simulink model "TaliRo_monitoring_subsytem"  (R2019b)
settings: Solver=VariableStepAuto  StartTime=0.0  StopTime=10.0  RelTol=1e-3
undefined symbols (not defined in the file): nb_rooms, nb_step_to_fifteen_min, nb_step_to_one_h, nb_step_to_thirty_min
libraries: S_TaLiRo x6, dspstat3 x6
settings Model: Creator=tong  LastModifiedBy=pat

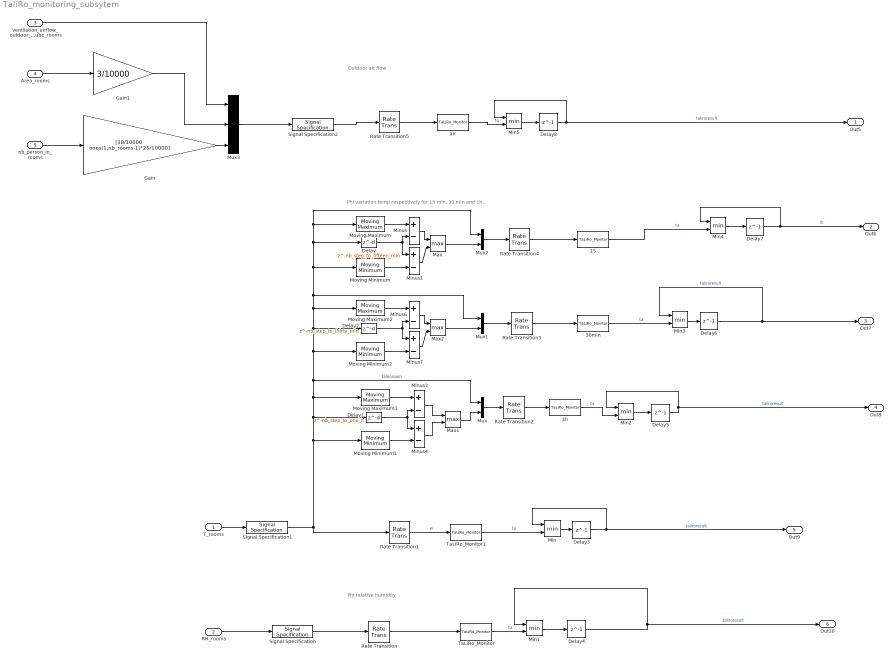
== system TaliRo_monitoring_subsytem ==
  note: Phi relative humidity
  note: Outdoor air flow
  note: Phi variation temp respectively for 15 min, 30 min and 1h.
  T_rooms : Inport  PortDimensions=nb_rooms
  RH_rooms : Inport  Port=2  PortDimensions=nb_rooms
  ventilation_airflow_outdoor_air_mcube_rooms : Inport  Port=3  PortDimensions=nb_rooms
  Area_rooms : Inport  Port=4  PortDimensions=nb_rooms
  nb_person_in_rooms : Inport  Port=5  OutDataTypeStr=double  PortDimensions=nb_rooms
  15 : S_TaLiRo/TaLiRo_Monitor  SFunctionModules=''
      settings: SourceProductName=S-TaLiRo
  1h : S_TaLiRo/TaLiRo_Monitor  SFunctionModules=''
      settings: SourceProductName=S-TaLiRo
  30min : S_TaLiRo/TaLiRo_Monitor  SFunctionModules=''
      settings: SourceProductName=S-TaLiRo
  Delay : Delay  DelayLength=nb_step_to_fifteen_min  InitialCondition=0
  Delay1 : Delay  DelayLength=nb_step_to_one_h  InitialCondition=0
  Delay2 : Delay  DelayLength=nb_step_to_thirty_min  InitialCondition=0
  Delay{3..8} (6 alike) : Delay  DelayLength=1  InitialCondition=0
  Gain : Gain  Gain=[38/10000 ones(1,nb_rooms-1)*25/10000]
  Gain1 : Gain  Gain=3/10000
  Max : MinMax  Function=max  Inputs=2
  Max1 : MinMax  Function=max  Inputs=2
  Max2 : MinMax  Function=max  Inputs=2
  Min{,1..5} (6 alike) : MinMax  Inputs=2
  Minus{,1,3..4,6..7} (6 alike) : Sum  Inputs=+-
  Moving Maximum : dspstat3/Moving Maximum  SpecifyWindowLength=on  WindowLength=nb_step_to_fifteen_min  SimulateUsing=Code generation
      settings: SourceProductName=DSP System Toolbox  SourceProductBaseCode=DS
  Moving Maximum1 : dspstat3/Moving Maximum  SpecifyWindowLength=on  WindowLength=nb_step_to_one_h  SimulateUsing=Code generation
      settings: SourceProductName=DSP System Toolbox  SourceProductBaseCode=DS
  Moving Maximum2 : dspstat3/Moving Maximum  SpecifyWindowLength=on  WindowLength=nb_step_to_thirty_min  SimulateUsing=Code generation
      settings: SourceProductName=DSP System Toolbox  SourceProductBaseCode=DS
  Moving Minimum : dspstat3/Moving Minimum  SpecifyWindowLength=on  WindowLength=nb_step_to_fifteen_min  SimulateUsing=Code generation
      settings: SourceProductName=DSP System Toolbox  SourceProductBaseCode=DS
  Moving Minimum1 : dspstat3/Moving Minimum  SpecifyWindowLength=on  WindowLength=nb_step_to_one_h  SimulateUsing=Code generation
      settings: SourceProductName=DSP System Toolbox  SourceProductBaseCode=DS
  Moving Minimum2 : dspstat3/Moving Minimum  SpecifyWindowLength=on  WindowLength=nb_step_to_thirty_min  SimulateUsing=Code generation
      settings: SourceProductName=DSP System Toolbox  SourceProductBaseCode=DS
  Mux : Mux  Inputs=2
  Mux1 : Mux  Inputs=2
  Mux2 : Mux  Inputs=2
  Mux3 : Mux  Inputs=[nb_rooms nb_rooms nb_rooms]
  Rate Transition{,1..5} (6 alike) : RateTransition  OutPortSampleTime=0.1
  Signal Specification : SignalSpecification  OutMin=-0.25  OutMax=1.25  Dimensions=nb_rooms
  Signal Specification1 : SignalSpecification  OutMin=-100  OutMax=100  Dimensions=nb_rooms
  Signal Specification2 : SignalSpecification  OutMin=-10000  OutMax=10000  Dimensions=nb_rooms*3
  TaLiRo_Monitor : S_TaLiRo/TaLiRo_Monitor  SFunctionModules=''
      settings: SourceProductName=S-TaLiRo
  TaLiRo_Monitor1 : S_TaLiRo/TaLiRo_Monitor  SFunctionModules=''
      settings: SourceProductName=S-TaLiRo
  air : S_TaLiRo/TaLiRo_Monitor  SFunctionModules=''
      settings: SourceProductName=S-TaLiRo
  Out5 : Outport
  Out6 : Outport  Port=2
  Out7 : Outport  Port=3
  Out8 : Outport  Port=4
  Out9 : Outport  Port=5
  Out10 : Outport  Port=6
  wires:
  Signal Specification/1 -> Rate Transition/1
  Minus1/1 -> Max/2
  T_rooms/1 -> Signal Specification1/1
  Moving Maximum2/1 -> Minus6/1
  Signal Specification1/1 -> Rate Transition1/1, Delay1/1, Mux/1, Mux1/1, Delay/1, Mux2/1, Moving Maximum/1, Moving Minimum/1, Moving Maximum2/1, Delay2/1, Moving Minimum2/1, Moving Maximum1/1, Moving Minimum1/1  "taliroroom"
  Max2/1 -> Mux1/2
  Max/1 -> Mux2/2
  Delay2/1 -> Minus6/2, Minus7/1
  Gain1/1 -> Mux3/2
  Area_rooms/1 -> Gain1/1
  Minus4/1 -> Max1/2
  Delay1/1 -> Minus3/2, Minus4/1
  nb_person_in_rooms/1 -> Gain/1
  Minus7/1 -> Max2/2
  Mux1/1 -> Rate Transition3/1
  Mux3/1 -> Signal Specification2/1
  RH_rooms/1 -> Signal Specification/1
  Gain/1 -> Mux3/3
  Minus/1 -> Max/1
  Moving Minimum2/1 -> Minus7/2
  Moving Minimum1/1 -> Minus4/2
  Moving Maximum/1 -> Minus/1
  Minus3/1 -> Max1/1
  Minus6/1 -> Max2/1
  Delay/1 -> Minus1/1, Minus/2
  Moving Maximum1/1 -> Minus3/1
  Mux2/1 -> Rate Transition4/1
  Max1/1 -> Mux/2
  Mux/1 -> Rate Transition2/1
  ventilation_airflow_outdoor_air_mcube_rooms/1 -> Mux3/1
  Moving Minimum/1 -> Minus1/2
  Rate Transition/1 -> TaLiRo_Monitor/1
  Rate Transition1/1 -> TaLiRo_Monitor1/1  "w"
  Rate Transition2/1 -> 1h/1
  Rate Transition3/1 -> 30min/1
  Rate Transition4/1 -> 15/1
  Min/1 -> Delay3/1
  Delay3/1 -> Min/1, Out9/1  "taliroresult"
  TaLiRo_Monitor1/1 -> Min/2  "ta"
  TaLiRo_Monitor/1 -> Min1/2  "ta"
  Min1/1 -> Delay4/1
  Delay4/1 -> Min1/1, Out10/1  "taliroresult"
  1h/1 -> Min2/2  "ta"
  Min2/1 -> Delay5/1
  Delay5/1 -> Out8/1, Min2/1  "taliroresult"
  30min/1 -> Min3/2  "ta"
  Min3/1 -> Delay6/1
  Delay6/1 -> Min3/1, Out7/1  "taliroresult"
  15/1 -> Min4/2  "ta"
  Min4/1 -> Delay7/1
  Delay7/1 -> Out6/1, Min4/1  "lt"
  Rate Transition5/1 -> air/1
  Signal Specification2/1 -> Rate Transition5/1
  air/1 -> Min5/2  "ta"
  Delay8/1 -> Min5/1, Out5/1  "taliroresult"
  Min5/1 -> Delay8/1
